simulink model "BF_Q1_ERP"  (R2025b)
settings: Solver=VariableStepAuto  StartTime=0.0  StopTime=2000  RelTol=1e-3
settings Model: Creator=Louis  LastModifiedBy=Louis

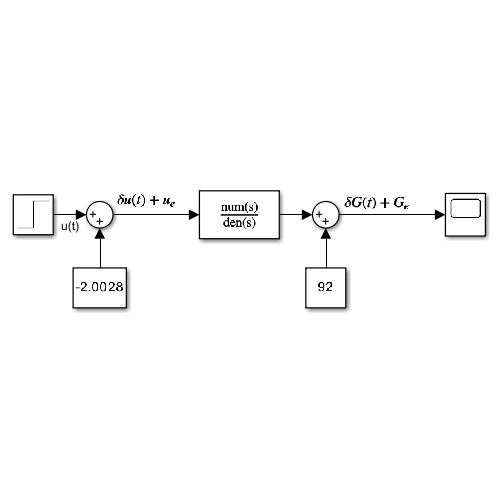
[thumbnail: Simulink's stored preview of the top-level diagram]
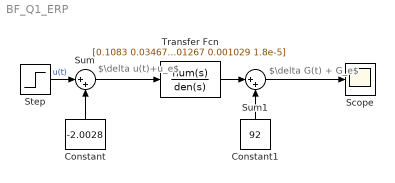
== system BF_Q1_ERP ==
  note: $\delta G(t) + G_e$
  note: $\delta u(t)+u_e$
  Constant : Constant  Value=-2.0028
  Constant1 : Constant  Value=92
  Scope : Scope
      settings: ActiveDisplayYMinimum=-1  ActiveDisplayYMaximum=1  DataLoggingVariableName=ERP  DataLoggingSaveFormat=Array
  Step : Step  Time=0  After=2  SampleTime=0
  Sum : Sum  Inputs=|++
  Sum1 : Sum  Inputs=|++
  Transfer Fcn : TransferFcn  Numerator=[0.1083 0.03467 -0.0003252 1.371e-23]  Denominator=[1 0.3315 0.01267 0.001029 1.8e-5]
  wires:
  Step/1 -> Sum/1  "u(t)"
  Sum/1 -> Transfer Fcn/1
  Constant/1 -> Sum/2
  Transfer Fcn/1 -> Sum1/1
  Constant1/1 -> Sum1/2
  Sum1/1 -> Scope/1
